simulink model "DYNctl_ver4_etud_decouple_Asserprof"  (R2014b)
settings: Solver=ode45  StartTime=0.0  StopTime=tfin  FixedStep=0.001  RelTol=1e-09
values from neighbouring files (symbols this model uses):
  C_plaque = [1 0 0]    [Decouplage.m]
  C_sphere = [1 0; 0 1]    [Decouplage.m]
  D_sphere = [0 0]'    [Decouplage.m]
  decoup_phi = [0 1 0; PP(1,1) 0 PC_11_eq; 0 0 CC(1,1)]    [Decouplage.m]
  decoup_phi_in = [0 0 CV(1,1)]'    [Decouplage.m]
  decoup_sp_x = [0 1;0 0]    [Decouplage.m]
  decoup_sp_x_in = [0 A(9,2)]'    [Decouplage.m]
  decoup_sp_y = [0 1;0 0]    [Decouplage.m]
  decoup_sp_y_in = [0 A(10,1)]'    [Decouplage.m]
  decoup_theta = [0 1 0; PP(2,2) 0 PC_22_eq; 0 0 CC(2,2)]    [Decouplage.m]
  decoup_theta_in = [0 0 CV(2,2)]'    [Decouplage.m]
  decoup_z = [0 1 0; PP(3,3) 0 PC_33_eq; 0 0 CC(3,3)]    [Decouplage.m]
  decoup_z_in = [0 0 CV(3,3)]'    [Decouplage.m]
  Kp_sphere = -0.705    [bancEssaiConstantes.m]
  Kv_sphere = -0.57085    [bancEssaiConstantes.m]
  phi_eq = 0    [MatlabEquilibre.m]    (also in equilibre.m)
  theta_eq = 0    [MatlabEquilibre.m]    (also in equilibre.m)
  v_sx_eq = 0    [MatlabEquilibre.m]
  v_sy_eq = 0    [MatlabEquilibre.m]
  Va_eq = R_bobine * Ia_eq    [MatlabEquilibre.m]    (also in bancessai_ini.m = Ia_eq*R_bobine; equilibre.m = Ia_eq*R_bobine)
  Vb_eq = R_bobine * Ib_eq    [MatlabEquilibre.m]    (also in bancessai_ini.m = Ib_eq*R_bobine; equilibre.m = Ib_eq*R_bobine)
  Vc_eq = R_bobine * Ic_eq    [MatlabEquilibre.m]    (also in bancessai_ini.m = Ic_eq*R_bobine; equilibre.m = Ic_eq*R_bobine)
  XD = r_DEF*sind(30)    [MatlabProjet.m]    (also in bancEssaiConstantes.m = +rDEF*sind(30); bancessai_ini.m; matrices_syms.m)
  XE = -r_DEF    (= -0.08)    [MatlabProjet.m]    (also in bancEssaiConstantes.m; bancessai_ini.m; matrices_syms.m)
  xs_eq = xs    (= 0)    [equilibre.m]
  YD = r_DEF*cosd(30)    [MatlabProjet.m]    (also in bancEssaiConstantes.m = +rDEF*cosd(30); bancessai_ini.m; matrices_syms.m)
  ys_eq = ys    (= 0)    [equilibre.m]
  Z0_eq = 0    [MatlabEquilibre.m]    (also in equilibre.m = 0.015)
undefined symbols (not defined in the file or in its folder): den_pt, den_z, num_pt, num_z, sym2poly
settings Model: Creator=delafontaine  LastModifiedBy=lemg2013
settings SolverCC: AlgebraicLoopSolver=LineSearch
settings DataIOCC: SignalLoggingSaveFormat=ModelDataLogs
settings DebuggingCC: UnderspecifiedInitializationDetection=Classic  MergeDetectMultiDrivingBlocksExec=none  SolverPrmCheckMsg=none  MultiTaskDSMMsg=warning  MultiTaskCondExecSysMsg=none  FrameProcessingCompatibilityMsg=error
settings RTWCC: IncludeERTFirstTime=on

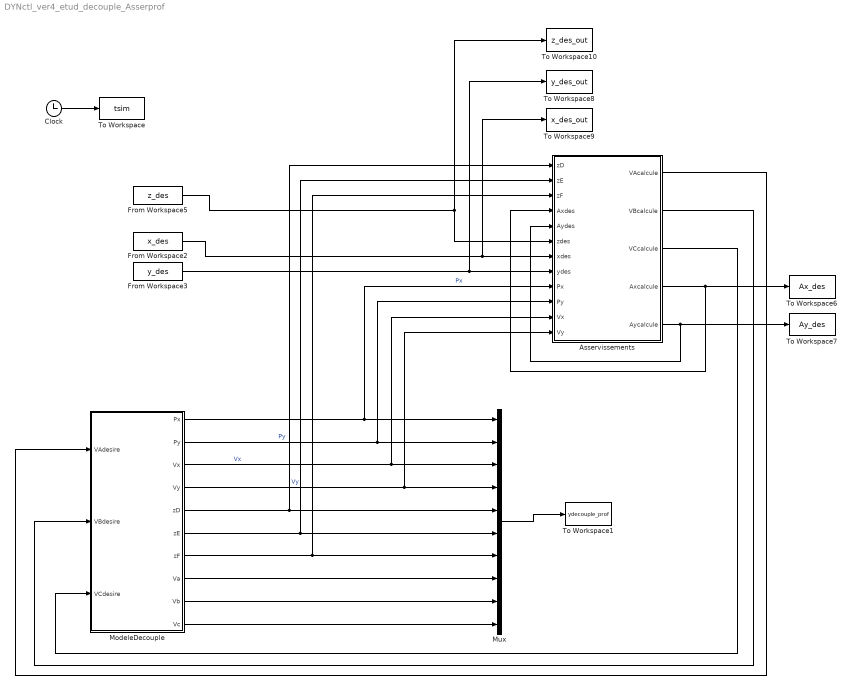
== system DYNctl_ver4_etud_decouple_Asserprof ==
  Asservissements : Subsystem
      mask help: Simulink:masks:GenSFuncDesc_MD
      mask Help: eval('feval(''rtwprivate'',''rtwhelpview'',''rtw_sfcn_block'')');
  Clock : Clock
  From Workspace2 : FromWorkspace  VariableName=x_des  SampleTime=0  Interpolate=off  OutputAfterFinalValue=Holding final value
  From Workspace3 : FromWorkspace  VariableName=y_des  SampleTime=0  Interpolate=off  OutputAfterFinalValue=Holding final value
  From Workspace5 : FromWorkspace  VariableName=z_des  SampleTime=0  Interpolate=off  OutputAfterFinalValue=Holding final value
  ModeleDecouple : Subsystem
      mask help: Simulink:masks:GenSFuncDesc_MD
      mask Help: eval('feval(''rtwprivate'',''rtwhelpview'',''rtw_sfcn_block'')');
  Mux : Mux  Inputs=10
  To Workspace : ToWorkspace  VariableName=tsim  SampleTime=-1
  To Workspace1 : ToWorkspace  VariableName=ydecouple_prof  SampleTime=-1
  To Workspace10 : ToWorkspace  VariableName=z_des_out  SampleTime=-1
  To Workspace6 : ToWorkspace  VariableName=Ax_des  SampleTime=-1
  To Workspace7 : ToWorkspace  VariableName=Ay_des  SampleTime=-1
  To Workspace8 : ToWorkspace  VariableName=y_des_out  SampleTime=-1
  To Workspace9 : ToWorkspace  VariableName=x_des_out  SampleTime=-1
  wires:
  Clock/1 -> To Workspace/1
  From Workspace5/1 -> Asservissements/6(zdes), To Workspace10/1
  ModeleDecouple/1(Px) -> Mux/1, Asservissements/9(Px)  "Px"
  ModeleDecouple/2(Py) -> Asservissements/10(Py), Mux/2  "Py"
  ModeleDecouple/3(Vx) -> Mux/3, Asservissements/11(Vx)  "Vx"
  ModeleDecouple/4(Vy) -> Asservissements/12(Vy), Mux/4  "Vy"
  From Workspace3/1 -> Asservissements/8(ydes), To Workspace8/1
  From Workspace2/1 -> Asservissements/7(xdes), To Workspace9/1
  ModeleDecouple/5(zD) -> Asservissements/1(zD), Mux/5
  ModeleDecouple/6(zE) -> Asservissements/2(zE), Mux/6
  ModeleDecouple/7(zF) -> Asservissements/3(zF), Mux/7
  Asservissements/4(Axcalcule) -> Asservissements/4(Axdes), To Workspace6/1
  Asservissements/5(Aycalcule) -> Asservissements/5(Aydes), To Workspace7/1
  Asservissements/1(VAcalcule) -> ModeleDecouple/1(VAdesire)
  Asservissements/2(VBcalcule) -> ModeleDecouple/2(VBdesire)
  Asservissements/3(VCcalcule) -> ModeleDecouple/3(VCdesire)
  Mux/1 -> To Workspace1/1
  ModeleDecouple/8(Va) -> Mux/8
  ModeleDecouple/9(Vb) -> Mux/9
  ModeleDecouple/10(Vc) -> Mux/10

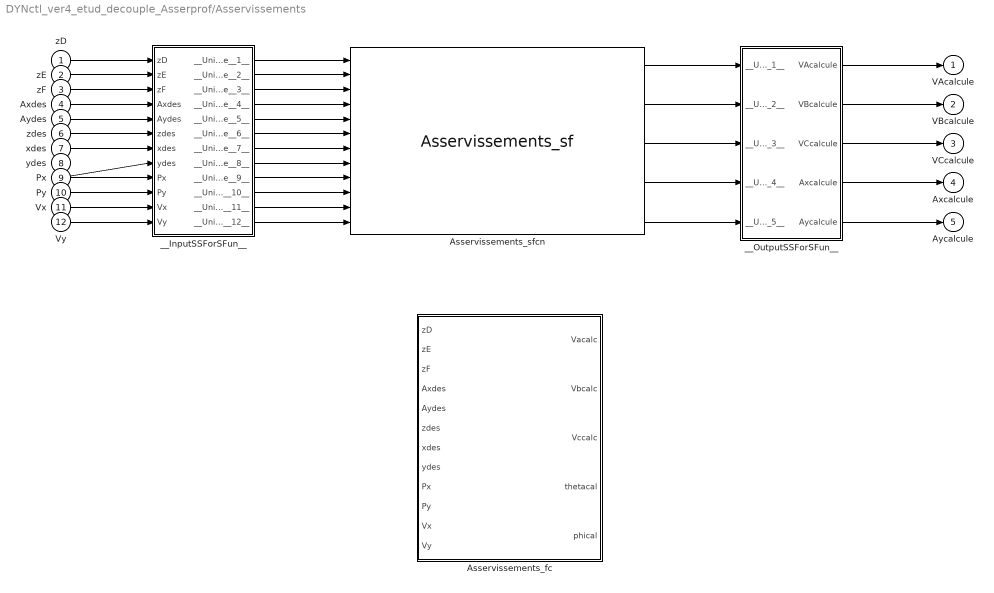
== system DYNctl_ver4_etud_decouple_Asserprof/Asservissements ==
  zD : Inport
  zE : Inport  Port=2
  zF : Inport  Port=3
  Axdes : Inport  Port=4
  Aydes : Inport  Port=5
  zdes : Inport  Port=6
  xdes : Inport  Port=7
  ydes : Inport  Port=8
  Px : Inport  Port=9
  Py : Inport  Port=10
  Vx : Inport  Port=11
  Vy : Inport  Port=12
  Asservissements_fc : Subsystem
  Asservissements_sfcn : S-Function  FunctionName=Asservissements_sf  SFunctionModules=""  EnableBusSupport=off  mask{rtw_sf_name=Asservissements_sf, showVar=off}
      mask prompts: rtw_sf_name "Simulink:masks:GenSFuncName_MP"; showVar "Simulink:masks:GenSFuncShowModuleList_MP"
      mask help: Simulink:masks:GenSFuncDesc_MD
      mask init:
      | displist = '';
      | if ~strcmp(get_param(gcb, 'FunctionName'), rtw_sf_name);
      |   set_param(gcb, 'FunctionName', rtw_sf_name);
      | end
      | % Check if we are generating code
      | rtw_mode = false;
      | if strcmpi(get_param(bdroot(gcb),'SimulationStatus'),'Initializing')
      | 	rtw_mode = strcmpi(get_param(bdroot(gcb),'BuildingRTWCode'),'on') && ...
      | 		~strcmpi(get_param(bdroot(gcb),'TargetStyle'),'SimulationTarget');
      | end
      | if showVar || rtw_mode
      | 	if exist('rtwsfunc') == 2 | exist('rtwsfunc') == 6
      | 		tmplist = rtwsfunc(rtw_sf_name,gcb);
      | 		tmplist = DAStudio.message('Simulink:masks:GenSFuncListOfModules_IC', tmplist);
      | 	elseif showVar
      | 		tmplist1 = DAStudio.message('Simulink:masks:GenSFuncListOfModules_IC', '');
      |         tmplist2 = DAStudio.message('Simulink:masks:GenSFuncNotLicensed_IC');
      |         tmplist = [tmplist1 tmplist2];
      |  	end
      | end
      | if showVar
      |   displist = tmplist;
      | end
      settings: CopyFcn=|
      | if ~strcmp(get_param(gcb,'Linkstatus'),'none') && ...
      | ~strcmp(get_param(gcb,'Linkstatus'),'implicit')
      |   set_param(gcb,'LinkStatus','none');
      | end
      mask Help: eval('feval(''rtwprivate'',''rtwhelpview'',''rtw_sfcn_block'')');
      mask Display:
      | port_label('input',1,'zD');
      | port_label('input',2,'zE');
      | port_label('input',3,'zF');
      | port_label('input',4,'Axdes');
      | port_label('input',5,'Aydes');
      | port_label('input',6,'zdes');
      | port_label('input',7,'xdes');
      | port_label('input',8,'ydes');
      | port_label('input',9,'Px');
      | port_label('input',10,'Py');
      | port_label('input',11,'Vx');
      | port_label('input',12,'Vy');
      | port_label('output',1,'VAcalcule');
      | port_label('output',2,'VBcalcule');
      | port_label('output',3,'VCcalcule');
      | port_label('output',4,'Axcalcule');
      | port_label('output',5,'Aycalcule');
  __InputSSForSFun__ : Subsystem
  __OutputSSForSFun__ : Subsystem
  VAcalcule : Outport
  VBcalcule : Outport  Port=2
  VCcalcule : Outport  Port=3
  Axcalcule : Outport  Port=4
  Aycalcule : Outport  Port=5
  wires:
  zD/1 -> __InputSSForSFun__/1(zD)
  zE/1 -> __InputSSForSFun__/2(zE)
  zF/1 -> __InputSSForSFun__/3(zF)
  Axdes/1 -> __InputSSForSFun__/4(Axdes)
  Aydes/1 -> __InputSSForSFun__/5(Aydes)
  zdes/1 -> __InputSSForSFun__/6(zdes)
  xdes/1 -> __InputSSForSFun__/7(xdes)
  ydes/1 -> __InputSSForSFun__/8(ydes)
  Px/1 -> __InputSSForSFun__/9(Px)
  Py/1 -> __InputSSForSFun__/10(Py)
  Vx/1 -> __InputSSForSFun__/11(Vx)
  Vy/1 -> __InputSSForSFun__/12(Vy)
  __InputSSForSFun__/1(__UniqueOutportName__1__) -> Asservissements_sfcn/1
  __InputSSForSFun__/2(__UniqueOutportName__2__) -> Asservissements_sfcn/2
  __InputSSForSFun__/3(__UniqueOutportName__3__) -> Asservissements_sfcn/3
  __InputSSForSFun__/4(__UniqueOutportName__4__) -> Asservissements_sfcn/4
  __InputSSForSFun__/5(__UniqueOutportName__5__) -> Asservissements_sfcn/5
  __InputSSForSFun__/6(__UniqueOutportName__6__) -> Asservissements_sfcn/6
  __InputSSForSFun__/7(__UniqueOutportName__7__) -> Asservissements_sfcn/7
  __InputSSForSFun__/8(__UniqueOutportName__8__) -> Asservissements_sfcn/8
  __InputSSForSFun__/9(__UniqueOutportName__9__) -> Asservissements_sfcn/9
  __InputSSForSFun__/10(__UniqueOutportName__10__) -> Asservissements_sfcn/10
  __InputSSForSFun__/11(__UniqueOutportName__11__) -> Asservissements_sfcn/11
  __InputSSForSFun__/12(__UniqueOutportName__12__) -> Asservissements_sfcn/12
  Asservissements_sfcn/1 -> __OutputSSForSFun__/1(__UniqueInportName__1__)
  Asservissements_sfcn/2 -> __OutputSSForSFun__/2(__UniqueInportName__2__)
  Asservissements_sfcn/3 -> __OutputSSForSFun__/3(__UniqueInportName__3__)
  Asservissements_sfcn/4 -> __OutputSSForSFun__/4(__UniqueInportName__4__)
  Asservissements_sfcn/5 -> __OutputSSForSFun__/5(__UniqueInportName__5__)
  __OutputSSForSFun__/1(VAcalcule) -> VAcalcule/1
  __OutputSSForSFun__/2(VBcalcule) -> VBcalcule/1
  __OutputSSForSFun__/3(VCcalcule) -> VCcalcule/1
  __OutputSSForSFun__/4(Axcalcule) -> Axcalcule/1
  __OutputSSForSFun__/5(Aycalcule) -> Aycalcule/1

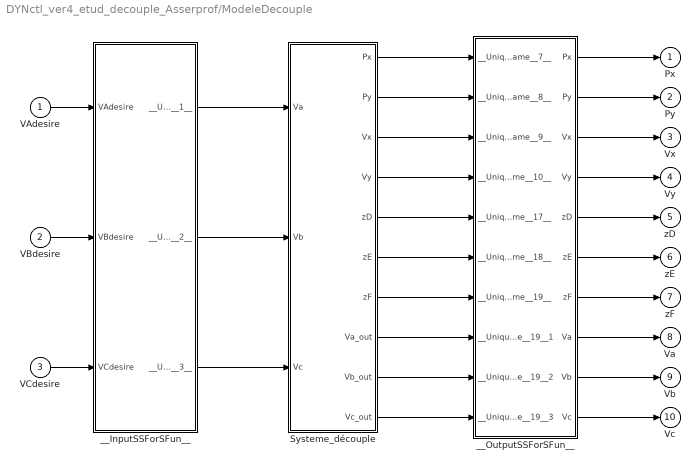
== system DYNctl_ver4_etud_decouple_Asserprof/ModeleDecouple ==
  VAdesire : Inport
  VBdesire : Inport  Port=2
  VCdesire : Inport  Port=3
  Systeme_découple : Subsystem
  __InputSSForSFun__ : Subsystem
  __OutputSSForSFun__ : Subsystem
  Px : Outport
  Py : Outport  Port=2
  Vx : Outport  Port=3
  Vy : Outport  Port=4
  zD : Outport  Port=5
  zE : Outport  Port=6
  zF : Outport  Port=7
  Va : Outport  Port=8
  Vb : Outport  Port=9
  Vc : Outport  Port=10
  wires:
  VAdesire/1 -> __InputSSForSFun__/1(VAdesire)
  VBdesire/1 -> __InputSSForSFun__/2(VBdesire)
  VCdesire/1 -> __InputSSForSFun__/3(VCdesire)
  __InputSSForSFun__/1(__UniqueOutportName__1__) -> Systeme_découple/1(Va)
  __OutputSSForSFun__/1(Px) -> Px/1
  __OutputSSForSFun__/2(Py) -> Py/1
  __OutputSSForSFun__/3(Vx) -> Vx/1
  __OutputSSForSFun__/4(Vy) -> Vy/1
  __OutputSSForSFun__/5(zD) -> zD/1
  __OutputSSForSFun__/6(zE) -> zE/1
  __OutputSSForSFun__/7(zF) -> zF/1
  __InputSSForSFun__/2(__UniqueOutportName__2__) -> Systeme_découple/2(Vb)
  __InputSSForSFun__/3(__UniqueOutportName__3__) -> Systeme_découple/3("Vc ")
  __OutputSSForSFun__/8(Va) -> Va/1
  __OutputSSForSFun__/9(Vb) -> Vb/1
  __OutputSSForSFun__/10(Vc) -> Vc/1
  Systeme_découple/5(zD) -> __OutputSSForSFun__/5(__UniqueInportName__17__)
  Systeme_découple/6(zE) -> __OutputSSForSFun__/6(__UniqueInportName__18__)
  Systeme_découple/7(zF) -> __OutputSSForSFun__/7(__UniqueInportName__19__)
  Systeme_découple/8(Va_out) -> __OutputSSForSFun__/8(__UniqueInportName__19__1)
  Systeme_découple/9(Vb_out) -> __OutputSSForSFun__/9(__UniqueInportName__19__2)
  Systeme_découple/10(Vc_out) -> __OutputSSForSFun__/10(__UniqueInportName__19__3)
  Systeme_découple/1(Px) -> __OutputSSForSFun__/1(__UniqueInportName__7__)
  Systeme_découple/2(Py) -> __OutputSSForSFun__/2(__UniqueInportName__8__)
  Systeme_découple/4(Vy) -> __OutputSSForSFun__/4(__UniqueInportName__10__)
  Systeme_découple/3(Vx) -> __OutputSSForSFun__/3(__UniqueInportName__9__)

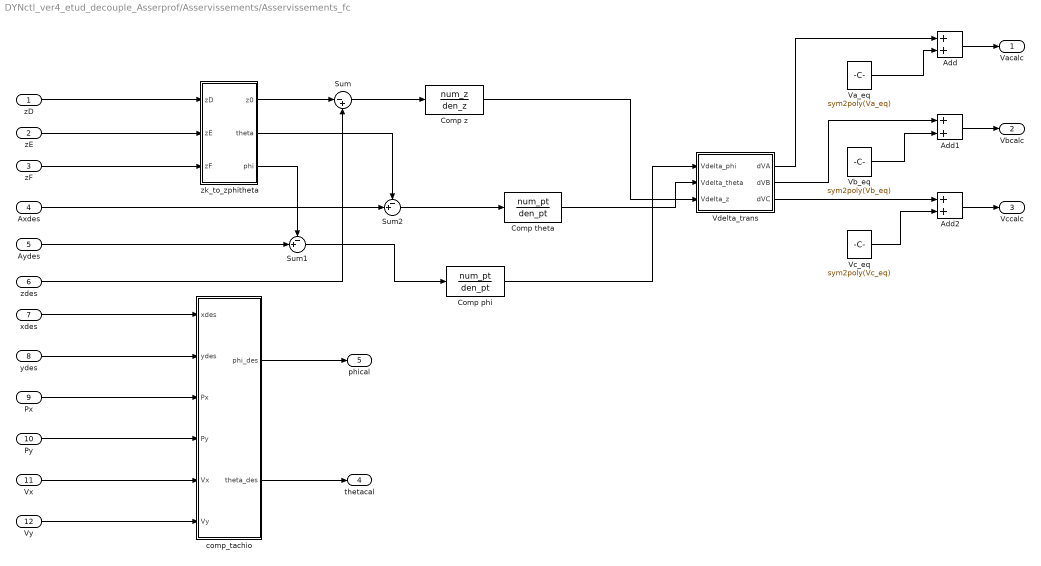
== system DYNctl_ver4_etud_decouple_Asserprof/Asservissements/Asservissements_fc ==
  zD : Inport
  zE : Inport  Port=2
  zF : Inport  Port=3
  Axdes : Inport  Port=4
  Aydes : Inport  Port=5
  zdes : Inport  Port=6
  xdes : Inport  Port=7
  ydes : Inport  Port=8
  Px : Inport  Port=9
  Py : Inport  Port=10
  Vx : Inport  Port=11
  Vy : Inport  Port=12
  Add : Sum
  Add1 : Sum
  Add2 : Sum
  Comp phi : TransferFcn  Numerator=num_pt  Denominator=den_pt
  Comp theta : TransferFcn  Numerator=num_pt  Denominator=den_pt
  Comp z : TransferFcn  Numerator=num_z  Denominator=den_z
  Sum : Sum  Inputs=|-+
  Sum1 : Sum  Inputs=-+|
  Sum2 : Sum  Inputs=-+|
  Va_eq : Constant  Value=sym2poly(Va_eq)  VectorParams1D=off
  Vb_eq : Constant  Value=sym2poly(Vb_eq)  VectorParams1D=off
  Vc_eq : Constant  Value=sym2poly(Vc_eq)  VectorParams1D=off
  Vdelta_trans : Subsystem
  comp_tachio : Subsystem
  zk_to_zphitheta : Subsystem
  Vacalc : Outport
  Vbcalc : Outport  Port=2
  Vccalc : Outport  Port=3
  thetacal : Outport  Port=4
  phical : Outport  Port=5
  wires:
  zD/1 -> zk_to_zphitheta/1(zD)
  zE/1 -> zk_to_zphitheta/2(zE)
  zF/1 -> zk_to_zphitheta/3(zF)
  zdes/1 -> Sum/2
  zk_to_zphitheta/1(z0) -> Sum/1
  Sum/1 -> Comp z/1
  Comp z/1 -> Vdelta_trans/3(Vdelta_z)
  xdes/1 -> comp_tachio/1(xdes)
  ydes/1 -> comp_tachio/2(ydes)
  Px/1 -> comp_tachio/3(Px)
  Py/1 -> comp_tachio/4(Py)
  Vx/1 -> comp_tachio/5(Vx)
  Vy/1 -> comp_tachio/6(Vy)
  comp_tachio/1(phi_des) -> phical/1
  zk_to_zphitheta/3(phi) -> Sum1/1
  comp_tachio/2(theta_des) -> thetacal/1
  zk_to_zphitheta/2(theta) -> Sum2/1
  Aydes/1 -> Sum1/2
  Axdes/1 -> Sum2/2
  Vdelta_trans/3(dVC) -> Add2/1
  Sum1/1 -> Comp phi/1
  Sum2/1 -> Comp theta/1
  Comp phi/1 -> Vdelta_trans/1(Vdelta_phi)
  Vdelta_trans/1(dVA) -> Add/1
  Vdelta_trans/2(dVB) -> Add1/1
  Comp theta/1 -> Vdelta_trans/2(Vdelta_theta)
  Add/1 -> Vacalc/1
  Add1/1 -> Vbcalc/1
  Add2/1 -> Vccalc/1
  Va_eq/1 -> Add/2
  Vc_eq/1 -> Add2/2
  Vb_eq/1 -> Add1/2

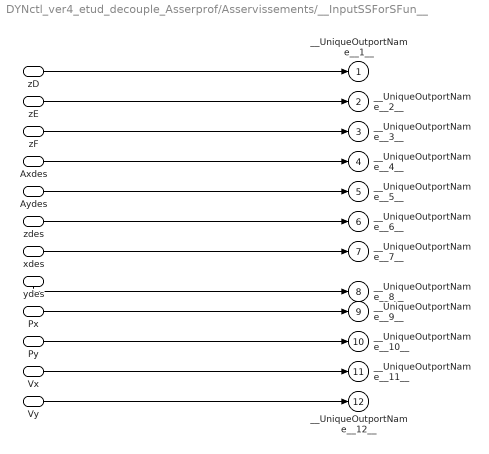
== system DYNctl_ver4_etud_decouple_Asserprof/Asservissements/__InputSSForSFun__ ==
  zD : Inport
  zE : Inport  Port=2
  zF : Inport  Port=3
  Axdes : Inport  Port=4
  Aydes : Inport  Port=5
  zdes : Inport  Port=6
  xdes : Inport  Port=7
  ydes : Inport  Port=8
  Px : Inport  Port=9
  Py : Inport  Port=10
  Vx : Inport  Port=11
  Vy : Inport  Port=12
  __UniqueOutportName__1__ : Outport
  __UniqueOutportName__2__ : Outport  Port=2
  __UniqueOutportName__3__ : Outport  Port=3
  __UniqueOutportName__4__ : Outport  Port=4
  __UniqueOutportName__5__ : Outport  Port=5
  __UniqueOutportName__6__ : Outport  Port=6
  __UniqueOutportName__7__ : Outport  Port=7
  __UniqueOutportName__8__ : Outport  Port=8
  __UniqueOutportName__9__ : Outport  Port=9
  __UniqueOutportName__10__ : Outport  Port=10
  __UniqueOutportName__11__ : Outport  Port=11
  __UniqueOutportName__12__ : Outport  Port=12
  wires:
  zD/1 -> __UniqueOutportName__1__/1
  zE/1 -> __UniqueOutportName__2__/1
  zF/1 -> __UniqueOutportName__3__/1
  Axdes/1 -> __UniqueOutportName__4__/1
  Aydes/1 -> __UniqueOutportName__5__/1
  zdes/1 -> __UniqueOutportName__6__/1
  xdes/1 -> __UniqueOutportName__7__/1
  ydes/1 -> __UniqueOutportName__8__/1
  Px/1 -> __UniqueOutportName__9__/1
  Py/1 -> __UniqueOutportName__10__/1
  Vx/1 -> __UniqueOutportName__11__/1
  Vy/1 -> __UniqueOutportName__12__/1

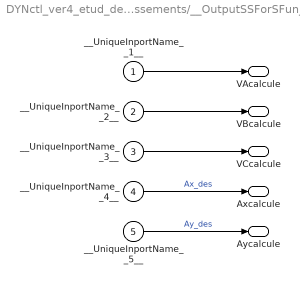
== system DYNctl_ver4_etud_decouple_Asserprof/Asservissements/__OutputSSForSFun__ ==
  __UniqueInportName__1__ : Inport
  __UniqueInportName__2__ : Inport  Port=2
  __UniqueInportName__3__ : Inport  Port=3
  __UniqueInportName__4__ : Inport  Port=4
  __UniqueInportName__5__ : Inport  Port=5
  VAcalcule : Outport
  VBcalcule : Outport  Port=2
  VCcalcule : Outport  Port=3
  Axcalcule : Outport  Port=4
  Aycalcule : Outport  Port=5
  wires:
  __UniqueInportName__1__/1 -> VAcalcule/1
  __UniqueInportName__2__/1 -> VBcalcule/1
  __UniqueInportName__3__/1 -> VCcalcule/1
  __UniqueInportName__4__/1 -> Axcalcule/1  "Ax_des"
  __UniqueInportName__5__/1 -> Aycalcule/1  "Ay_des"

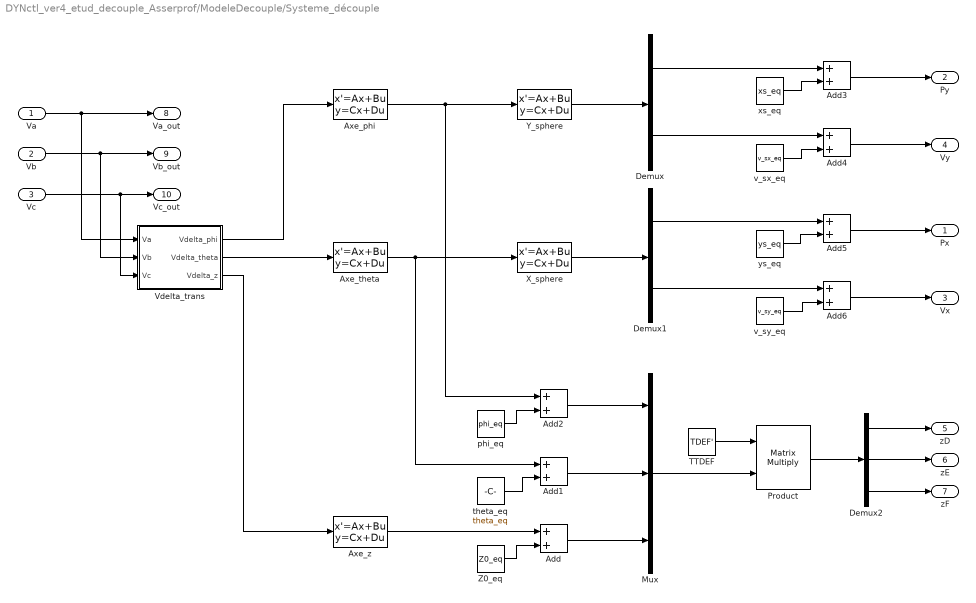
== system DYNctl_ver4_etud_decouple_Asserprof/ModeleDecouple/Systeme_découple ==
  Va : Inport
  Vb : Inport  Port=2
  "Vc " : Inport  Port=3
  Add{,1..6} (7 alike) : Sum
  Axe_phi : StateSpace  A=decoup_phi  B=decoup_phi_in  C=C_plaque  D=0  X0=0
  Axe_theta : StateSpace  A=decoup_theta  B=decoup_theta_in  C=C_plaque  D=0  X0=0
  Axe_z : StateSpace  A=decoup_z  B=decoup_z_in  C=C_plaque  D=0  X0=0
  Demux : Demux  Outputs=2
  Demux1 : Demux  Outputs=2
  Demux2 : Demux  Outputs=3
  Mux : Mux  Inputs=3
  Product : Product  Multiplication=Matrix(*)
  TTDEF : Constant  Value=TDEF'
  Vdelta_trans : Subsystem
  X_sphere : StateSpace  A=decoup_sp_x  B=decoup_sp_x_in  C=C_sphere  D=D_sphere  X0=0
  Y_sphere : StateSpace  A=decoup_sp_y  B=decoup_sp_y_in  C=C_sphere  D=D_sphere  X0=0
  Z0_eq : Constant  Value=Z0_eq
  phi_eq : Constant  Value=phi_eq
  theta_eq : Constant  Value=theta_eq
  v_sx_eq : Constant  Value=v_sx_eq
  v_sy_eq : Constant  Value=v_sy_eq
  xs_eq : Constant  Value=xs_eq
  ys_eq : Constant  Value=ys_eq
  Px : Outport
  Py : Outport  Port=2
  Vx : Outport  Port=3
  Vy : Outport  Port=4
  zD : Outport  Port=5
  zE : Outport  Port=6
  zF : Outport  Port=7
  Va_out : Outport  Port=8
  Vb_out : Outport  Port=9
  Vc_out : Outport  Port=10
  wires:
  Vb/1 -> Vb_out/1, Vdelta_trans/2(Vb)
  "Vc "/1 -> Vdelta_trans/3(Vc), Vc_out/1
  Vdelta_trans/1(Vdelta_phi) -> Axe_phi/1
  Vdelta_trans/2(Vdelta_theta) -> Axe_theta/1
  Vdelta_trans/3(Vdelta_z) -> Axe_z/1
  Axe_phi/1 -> Y_sphere/1, Add2/1
  Demux/2 -> Add4/1
  Demux/1 -> Add3/1
  Demux1/1 -> Add5/1
  Demux1/2 -> Add6/1
  xs_eq/1 -> Add3/2
  v_sx_eq/1 -> Add4/2
  ys_eq/1 -> Add5/2
  v_sy_eq/1 -> Add6/2
  phi_eq/1 -> Add2/2
  Add2/1 -> Mux/1
  Axe_theta/1 -> X_sphere/1, Add1/1
  theta_eq/1 -> Add1/2
  Add1/1 -> Mux/2
  Axe_z/1 -> Add/1
  Z0_eq/1 -> Add/2
  Add/1 -> Mux/3
  Add3/1 -> Py/1
  Add4/1 -> Vy/1
  Add5/1 -> Px/1
  Add6/1 -> Vx/1
  Demux2/1 -> zD/1
  Demux2/2 -> zE/1
  Demux2/3 -> zF/1
  TTDEF/1 -> Product/1
  Mux/1 -> Product/2
  Product/1 -> Demux2/1
  Y_sphere/1 -> Demux/1
  X_sphere/1 -> Demux1/1
  Va/1 -> Vdelta_trans/1(Va), Va_out/1

== system DYNctl_ver4_etud_decouple_Asserprof/ModeleDecouple/__InputSSForSFun__ ==
  VAdesire : Inport
  VBdesire : Inport  Port=2
  VCdesire : Inport  Port=3
  __UniqueOutportName__1__ : Outport
  __UniqueOutportName__2__ : Outport  Port=2
  __UniqueOutportName__3__ : Outport  Port=3
  wires:
  VAdesire/1 -> __UniqueOutportName__1__/1
  VBdesire/1 -> __UniqueOutportName__2__/1
  VCdesire/1 -> __UniqueOutportName__3__/1

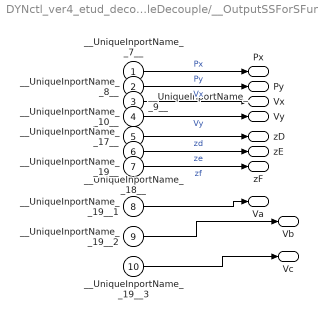
== system DYNctl_ver4_etud_decouple_Asserprof/ModeleDecouple/__OutputSSForSFun__ ==
  __UniqueInportName__7__ : Inport
  __UniqueInportName__8__ : Inport  Port=2
  __UniqueInportName__9__ : Inport  Port=3
  __UniqueInportName__10__ : Inport  Port=4
  __UniqueInportName__17__ : Inport  Port=5
  __UniqueInportName__18__ : Inport  Port=6
  __UniqueInportName__19__ : Inport  Port=7
  __UniqueInportName__19__1 : Inport  Port=8
  __UniqueInportName__19__2 : Inport  Port=9
  __UniqueInportName__19__3 : Inport  Port=10
  Px : Outport
  Py : Outport  Port=2
  Vx : Outport  Port=3
  Vy : Outport  Port=4
  zD : Outport  Port=5
  zE : Outport  Port=6
  zF : Outport  Port=7
  Va : Outport  Port=8
  Vb : Outport  Port=9
  Vc : Outport  Port=10
  wires:
  __UniqueInportName__7__/1 -> Px/1  "Px"
  __UniqueInportName__8__/1 -> Py/1  "Py"
  __UniqueInportName__9__/1 -> Vx/1  "Vx"
  __UniqueInportName__10__/1 -> Vy/1  "Vy"
  __UniqueInportName__17__/1 -> zD/1  "zd"
  __UniqueInportName__18__/1 -> zE/1  "ze"
  __UniqueInportName__19__/1 -> zF/1  "zf"
  __UniqueInportName__19__1/1 -> Va/1
  __UniqueInportName__19__2/1 -> Vb/1
  __UniqueInportName__19__3/1 -> Vc/1

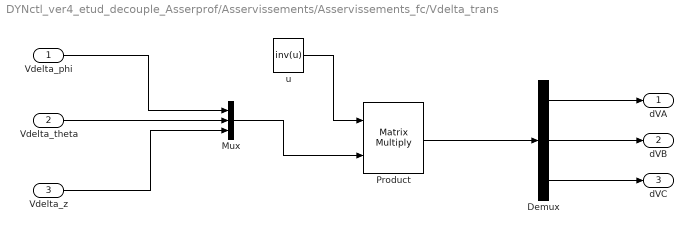
== system DYNctl_ver4_etud_decouple_Asserprof/Asservissements/Asservissements_fc/Vdelta_trans ==
  Vdelta_phi : Inport
  Vdelta_theta : Inport  Port=2
  Vdelta_z : Inport  Port=3
  Demux : Demux  Outputs=3
  Mux : Mux  Inputs=3
  Product : Product  Multiplication=Matrix(*)
  u : Constant  Value=inv(u)  VectorParams1D=off
  dVA : Outport
  dVB : Outport  Port=2
  dVC : Outport  Port=3
  wires:
  u/1 -> Product/1
  Mux/1 -> Product/2
  Demux/1 -> dVA/1
  Demux/2 -> dVB/1
  Demux/3 -> dVC/1
  Product/1 -> Demux/1
  Vdelta_phi/1 -> Mux/1
  Vdelta_theta/1 -> Mux/2
  Vdelta_z/1 -> Mux/3

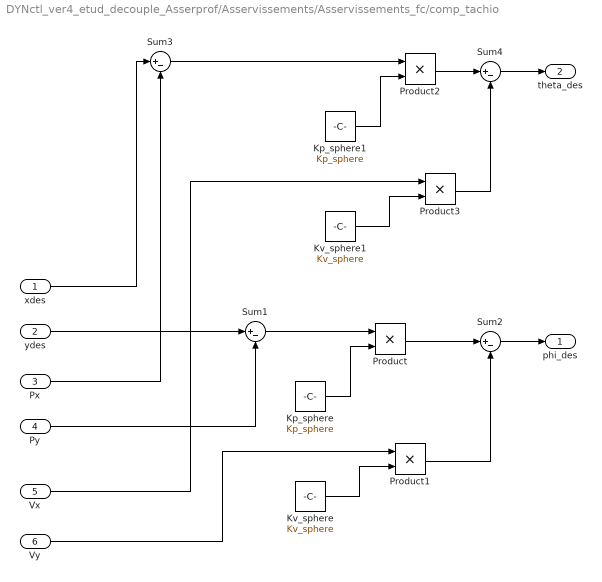
== system DYNctl_ver4_etud_decouple_Asserprof/Asservissements/Asservissements_fc/comp_tachio ==
  xdes : Inport
  ydes : Inport  Port=2
  Px : Inport  Port=3
  Py : Inport  Port=4
  Vx : Inport  Port=5
  Vy : Inport  Port=6
  Kp_sphere : Constant  Value=Kp_sphere
  Kp_sphere1 : Constant  Value=Kp_sphere
  Kv_sphere : Constant  Value=Kv_sphere
  Kv_sphere1 : Constant  Value=Kv_sphere
  Product{,1..3} (4 alike) : Product
  Sum{1..4} (4 alike) : Sum  Inputs=|+-
  phi_des : Outport
  theta_des : Outport  Port=2
  wires:
  ydes/1 -> Sum1/1
  Py/1 -> Sum1/2
  Sum1/1 -> Product/1
  Kp_sphere/1 -> Product/2
  Product/1 -> Sum2/1
  Product1/1 -> Sum2/2
  Vy/1 -> Product1/1
  Kv_sphere/1 -> Product1/2
  Sum2/1 -> phi_des/1
  xdes/1 -> Sum3/1
  Px/1 -> Sum3/2
  Sum3/1 -> Product2/1
  Kp_sphere1/1 -> Product2/2
  Product2/1 -> Sum4/1
  Product3/1 -> Sum4/2
  Vx/1 -> Product3/1
  Kv_sphere1/1 -> Product3/2
  Sum4/1 -> theta_des/1

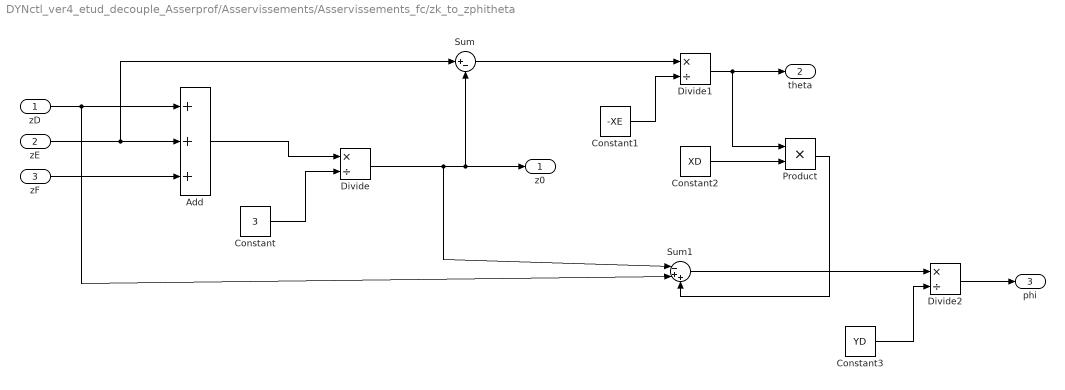
== system DYNctl_ver4_etud_decouple_Asserprof/Asservissements/Asservissements_fc/zk_to_zphitheta ==
  zD : Inport
  zE : Inport  Port=2
  zF : Inport  Port=3
  Add : Sum  Inputs=+++
  Constant : Constant  Value=3
  Constant1 : Constant  Value=-XE
  Constant2 : Constant  Value=XD
  Constant3 : Constant  Value=YD
  Divide : Product  Inputs=*/
  Divide1 : Product  Inputs=*/
  Divide2 : Product  Inputs=*/
  Product : Product
  Sum : Sum  Inputs=|+-
  Sum1 : Sum  Inputs=|-++
  z0 : Outport
  theta : Outport  Port=2
  phi : Outport  Port=3
  wires:
  zD/1 -> Sum1/2, Add/1
  zE/1 -> Sum/1, Add/2
  zF/1 -> Add/3
  Add/1 -> Divide/1
  Constant/1 -> Divide/2
  Divide/1 -> Sum1/1, Sum/2, z0/1
  Sum/1 -> Divide1/1
  Constant1/1 -> Divide1/2
  Divide1/1 -> Product/1, theta/1
  Constant2/1 -> Product/2
  Product/1 -> Sum1/3
  Sum1/1 -> Divide2/1
  Constant3/1 -> Divide2/2
  Divide2/1 -> phi/1

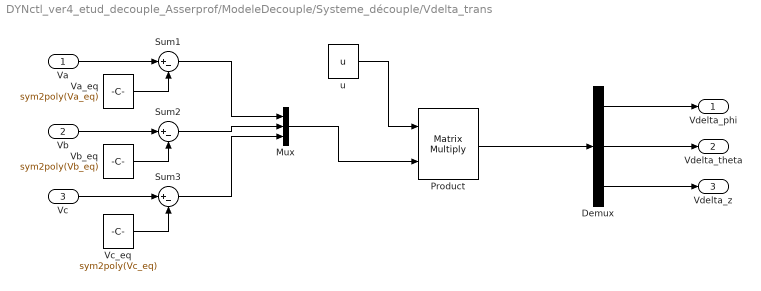
== system DYNctl_ver4_etud_decouple_Asserprof/ModeleDecouple/Systeme_découple/Vdelta_trans ==
  Va : Inport
  Vb : Inport  Port=2
  Vc : Inport  Port=3
  Demux : Demux  Outputs=3
  Mux : Mux  Inputs=3
  Product : Product  Multiplication=Matrix(*)
  Sum1 : Sum  Inputs=|+-
  Sum2 : Sum  Inputs=|+-
  Sum3 : Sum  Inputs=|+-
  Va_eq : Constant  Value=sym2poly(Va_eq)  VectorParams1D=off
  Vb_eq : Constant  Value=sym2poly(Vb_eq)  VectorParams1D=off
  Vc_eq : Constant  Value=sym2poly(Vc_eq)  VectorParams1D=off
  u : Constant  Value=u  VectorParams1D=off
  Vdelta_phi : Outport
  Vdelta_theta : Outport  Port=2
  Vdelta_z : Outport  Port=3
  wires:
  u/1 -> Product/1
  Mux/1 -> Product/2
  Demux/1 -> Vdelta_phi/1
  Demux/2 -> Vdelta_theta/1
  Demux/3 -> Vdelta_z/1
  Va/1 -> Sum1/1
  Vb/1 -> Sum2/1
  Vc/1 -> Sum3/1
  Product/1 -> Demux/1
  Sum1/1 -> Mux/1
  Sum2/1 -> Mux/2
  Sum3/1 -> Mux/3
  Va_eq/1 -> Sum1/2
  Vb_eq/1 -> Sum2/2
  Vc_eq/1 -> Sum3/2
